simulink model "Kalman_from_SSP"  (R2020a)
settings: Solver=VariableStepAuto  StartTime=0.0  StopTime=5  RelTol=1e-3
InitFcn:
  | load Data_motor_sine
undefined symbols (not defined in the file): An, Bn, Ln, Ts
settings Model: Creator=ramezani  LastModifiedBy=Artis
settings DataIOCC: ReturnWorkspaceOutputs=off
settings DebuggingCC: ArithmeticOperatorsInVariantConditions=warning
settings SFSimCC: CustomCodeUndefinedFunction=UseInterfaceOnly

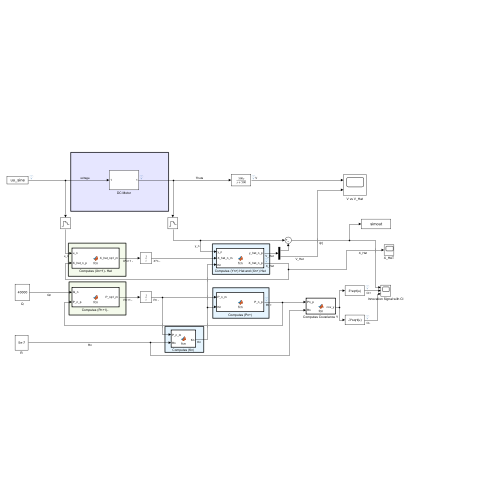
[thumbnail: Simulink's stored preview of the top-level diagram]
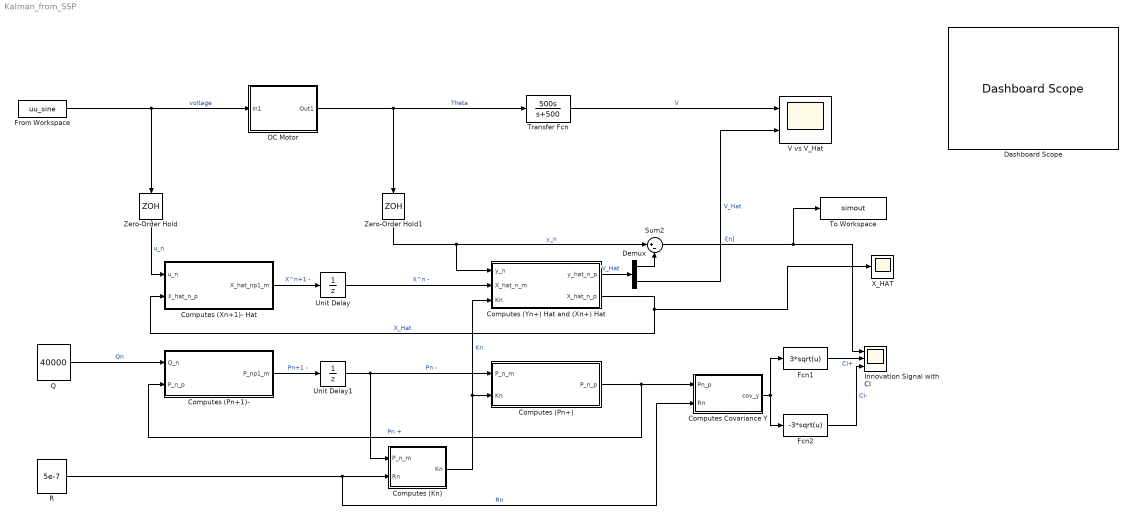
== system Kalman_from_SSP ==
  Computes (Kn) : MATLAB Function  TreatAsAtomicUnit=on
  Computes (Pn+) : MATLAB Function  TreatAsAtomicUnit=on
  "Computes (Pn+1)- " : MATLAB Function  TreatAsAtomicUnit=on
  Computes (Xn+1)- Hat : MATLAB Function  TreatAsAtomicUnit=on
  Computes (Yn+) Hat and (Xn+) Hat : MATLAB Function  TreatAsAtomicUnit=on
  Computes Covariance Y : MATLAB Function  TreatAsAtomicUnit=on
  DC Motor : Subsystem
  Dashboard Scope : DashboardScope
  Demux : Demux  Outputs=2
  Fcn1 : Fcn  Expr=3*sqrt(u)
  Fcn2 : Fcn  Expr=-3*sqrt(u)
  From Workspace : FromWorkspace  VariableName=uu_sine
  Innovation Signal with CI : Scope  NumInputPorts=3
  Q : Constant  Value=40000
  R : Constant  Value=5e-7
  Sum2 : Sum  Inputs=|+-
  To Workspace : ToWorkspace  VariableName=simout  SaveFormat=Timeseries  SampleTime=-1
  Transfer Fcn : TransferFcn  Numerator=[500 0]  Denominator=[1 500]
  Unit Delay : UnitDelay  InitialCondition=[0;0]  SampleTime=Ts  HasFrameUpgradeWarning=on
  Unit Delay1 : UnitDelay  InitialCondition=1*[.1 0;0 .1]  SampleTime=Ts  HasFrameUpgradeWarning=on
  V vs V_Hat : Scope  NumInputPorts=2
  X_HAT : Scope
  Zero-Order Hold : ZeroOrderHold  SampleTime=-1
  Zero-Order Hold1 : ZeroOrderHold  SampleTime=Ts
  wires:
  From Workspace/1 -> DC Motor/1(In1), Zero-Order Hold/1  "voltage"
  DC Motor/1(Out1) -> Transfer Fcn/1, Zero-Order Hold1/1  "Theta"
  Transfer Fcn/1 -> V vs V_Hat/1  "V"
  Zero-Order Hold/1 -> Computes (Xn+1)- Hat/1(u_n)  "u_n"
  Q/1 -> "Computes (Pn+1)- "/1(Q_n)  "Qn"
  Computes (Pn+)/1(P_n_p) -> Computes Covariance Y/1(Pn_p), "Computes (Pn+1)- "/2(P_n_p)  "Pn +"
  R/1 -> Computes (Kn)/2(Rn), Computes Covariance Y/2(Rn)  "Rn"
  Computes (Xn+1)- Hat/1(X_hat_np1_m) -> Unit Delay/1  "X^n+1 -"
  Unit Delay1/1 -> Computes (Pn+)/1(P_n_m), Computes (Kn)/1(P_n_m)  "Pn -"
  Unit Delay/1 -> Computes (Yn+) Hat and (Xn+) Hat/2(X_hat_n_m)  "X^n -"
  Computes (Yn+) Hat and (Xn+) Hat/1(y_hat_n_p) -> Demux/1  "V_Hat"
  Computes (Yn+) Hat and (Xn+) Hat/2(X_hat_n_p) -> X_HAT/1, Computes (Xn+1)- Hat/2(X_hat_n_p)  "X_Hat"
  "Computes (Pn+1)- "/1(P_np1_m) -> Unit Delay1/1  "Pn+1 -"
  Computes (Kn)/1(Kn) -> Computes (Yn+) Hat and (Xn+) Hat/3(Kn), Computes (Pn+)/2(Kn)  "Kn"
  Fcn1/1 -> Innovation Signal with CI/2  "CI+"
  Sum2/1 -> To Workspace/1, Innovation Signal with CI/1  "i[n]"
  Zero-Order Hold1/1 -> Computes (Yn+) Hat and (Xn+) Hat/1(y_n), Sum2/1  "y_n"
  Fcn2/1 -> Innovation Signal with CI/3  "CI-"
  Computes Covariance Y/1(cov_y) -> Fcn1/1, Fcn2/1
  Demux/2 -> V vs V_Hat/2  "V_Hat"
  Demux/1 -> Sum2/2

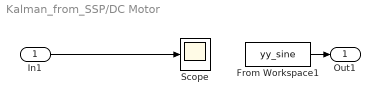
== system Kalman_from_SSP/DC Motor ==
  In1 : Inport
  From Workspace1 : FromWorkspace  VariableName=yy_sine
  Scope : Scope
  Out1 : Outport  VectorParamsAs1DForOutWhenUnconnected=off
  wires:
  From Workspace1/1 -> Out1/1
  In1/1 -> Scope/1

== matlab function Kalman_from_SSP/Computes (Yn+) Hat and (Xn+) Hat ==
  data: y_hat_n_p output; y_n input; X_hat_n_m input; X_hat_n_p output; Kn input; Hn parameter
function [y_hat_n_p,X_hat_n_p] = fcn(y_n,X_hat_n_m,Kn,Hn)
X_hat_n_p=X_hat_n_m+Kn*(y_n-Hn*X_hat_n_m);

y_hat_n_p=X_hat_n_p;

== matlab function Kalman_from_SSP/Computes (Xn+1)- Hat ==
  data: u_n input; X_hat_n_p input; X_hat_np1_m output; An parameter; Bn parameter
function X_hat_np1_m = fcn(u_n,X_hat_n_p, An, Bn)

X_hat_np1_m= An*X_hat_n_p + Bn*u_n;

== matlab function Kalman_from_SSP/Computes (Pn+1)-  ==
  data: Q_n input; P_n_p input; P_np1_m output; An parameter; Ln parameter
function P_np1_m = fcn(Q_n,P_n_p,An, Ln)

P_np1_m = An*P_n_p*An' + Ln*Q_n*Ln';

== matlab function Kalman_from_SSP/Computes (Pn+) ==
  data: P_n_m input; P_n_p output; Kn input; Hn parameter
function P_n_p = fcn(P_n_m,Kn,Hn)
P_n_p=P_n_m-Kn*Hn*P_n_m;

== matlab function Kalman_from_SSP/Computes (Kn) ==
  data: P_n_m input; Kn output; Rn input; Hn parameter
function Kn = fcn(P_n_m,Rn,Hn)

Kn=P_n_m*Hn'/(Hn*P_n_m*Hn'+Rn);

== matlab function Kalman_from_SSP/Computes Covariance Y ==
  data: Pn_p input; cov_y output; Rn input; Hn parameter
function cov_y = fcn(Pn_p,Rn, Hn)

cov_y= Hn * Pn_p * Hn'+ Rn;
